simulink model "FrequencySupport_OSC1_or_OSC2"  (R2022a)
settings: Solver=ode15s  StartTime=0.0  StopTime=50  RelTol=1e-3
model workspace (MAT data in the model file):
  Cdc = 0.05
  c_dc = 0.05
values from neighbouring files (symbols this model uses):
  P_dis_bat = [9604.62056476 1369.7268469 1306.14940083 1303.28868815 1261.92740103 1202.52269752 1169.74670515 1107.03788784 1057.53947406 962.184427064 965.562157323 899.489129709 ... (3456 elements, 1152x3)]    [result_base.mat]
undefined symbols (not defined in the file or in its folder): C, D, f0, H_rec, H_send, Hvirt_BES, Hvirt_PV, K_bat_vir, Kf_BES, Kf_dc, Kf_EL, Kf_PV, Kf_WT, OC_HVDC, P_EL_0, P_load_vsc_rec, P_load_vsc_rec_2, P_PV_0, P_send_0, P_WT_0, Pdc0, R_down_bat, R_down_EL, R_down_PV, R_down_WT, R_PV_up_req, R_syn_rec, R_up_bat, R_up_EL, R_up_PV, R_up_WT, R_WT_up_req, S_BES, S_EL, S_HVDC, S_PV, S_rec, S_rec_hydra, S_rec_syn, S_send, S_send_syn, S_WT, Sliding_window_t, T_ch, T_g_syn, T_g_w, T_rh, T_w
settings Model: Creator=Douzi  LastModifiedBy=Douzi

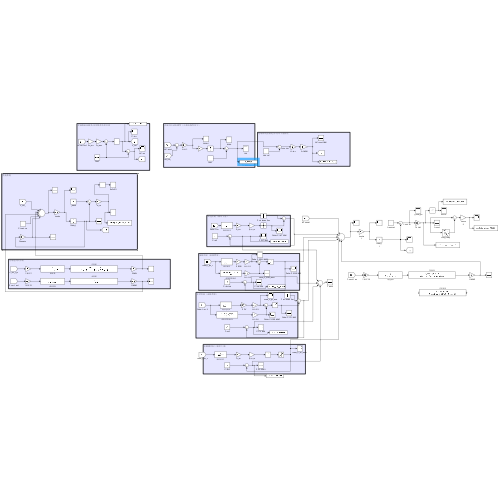
[thumbnail: Simulink's stored preview of the top-level diagram]
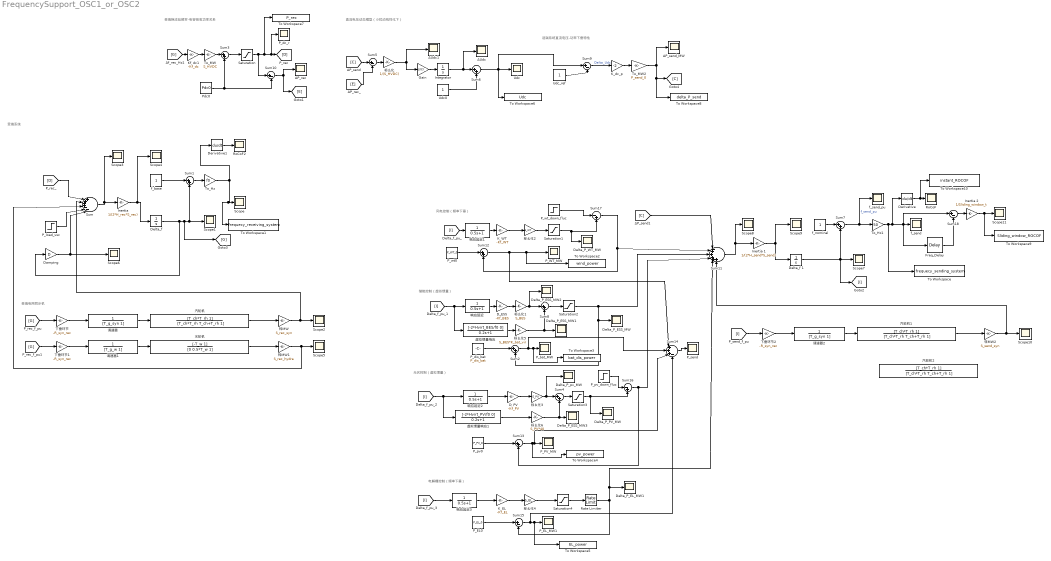
== system FrequencySupport_OSC1_or_OSC2 ==
  note: 受端电网同步机
  note: 储能控制（虚拟惯量）
  note: 风电控制（频率下垂）
  note: 受端换流站频率-电容吸收功率关系
  note: 受端系统
  note: 光伏控制（虚拟惯量）
  note: 电解槽控制（频率下垂）
  note: 直流电压动态模型（小扰动线性化下）
  note: 送端系统直流电压-功率下垂特性
  D_ESS : Gain  Gain=-Kf_BES
  D_PV : Gain  Gain=-Kf_PV
  Damping : Gain  Gain=D
  Delta_P_EL_MW1 : Scope
  Delta_P_ESS_MW{,1..3} (4 alike) : Scope
  Delta_P_PV_MW : Scope
  Delta_P_WT_MW : Scope
  Delta_P_pv_MW : Scope
  "Delta_f " : Integrator
  Delta_f 1 : Integrator
  Derivative : Derivative
  Derivative1 : Derivative
  Freq_Delay : TransportDelay  DelayTime=Sliding_window_t  InitialOutput=50
  Gain : Gain  Gain=1/(C)
  "Inertia " : Gain  Gain=1/(2*H_rec*S_rec)
  Inertia 1 : Gain  Gain=1/(2*H_send*S_send)
  Inertia 2 : Gain  Gain=1/Sliding_window_t
  Integrator : Integrator
  K_EL : Gain  Gain=-Kf_EL
  K_WT : Gain  Gain=-Kf_WT
  K_dc_p : Gain  Gain=-2
  Kf_dc1 : Gain  Gain=-Kf_dc
  P_EL0 : Constant  Value=P_EL_0
  P_EL_MW1 : Scope
  P_PV_MW : Scope
  P_WT_MW : Scope
  P_bat_MW : Scope
  P_dc_r : Scope
  P_dis_bat : Constant  Value=P_dis_bat
  P_load_vsc : Step  Before=P_load_vsc_rec  After=P_load_vsc_rec_2  SampleTime=0
  P_pv0 : Constant  Value=P_PV_0
  P_pv_down_fluc : Step  After=R_PV_up_req  SampleTime=0
  P_send : Scope
  P_wt0 : Constant  Value=P_WT_0
  P_wt_down_fluc : Step  After=R_WT_up_req  SampleTime=0
  Pdc0 : Constant  Value=Pdc0
  Rate Limiter : RateLimiter  RisingSlewLimit=0.2*S_EL  FallingSlewLimit=-0.2*S_EL  SampleTimeMode=inherited
  RoCoF : Scope
  RoCoF2 : Scope
  Saturation : Saturate  UpperLimit=S_HVDC*OC_HVDC  LowerLimit=0
  Saturation1 : Saturate  UpperLimit=R_up_WT  LowerLimit=-R_down_WT
  Saturation2 : Saturate  UpperLimit=R_up_bat  LowerLimit=-R_down_bat
  Saturation3 : Saturate  UpperLimit=R_up_PV  LowerLimit=-R_down_PV
  Saturation4 : Saturate  UpperLimit=R_up_EL  LowerLimit=-R_down_EL
  Scope{,1..11} (12 alike) : Scope
  Sum : Sum  Inputs=|++++--|
  Sum{1..4,6..8,12..13} (9 alike) : Sum  Inputs=|++
  Sum{5,9..10,15,18} (5 alike) : Sum  Inputs=|+-
  Sum11 : Sum  Inputs=|-+++++
  Sum14 : Sum  Inputs=|+++-
  Sum16 : Sum  Inputs=|-+
  Sum17 : Sum  Inputs=|-+
  To Workspace : ToWorkspace  VariableName=frequecy_sending_system  SaveFormat=Structure With Time  SampleTime=-1
  To Workspace1 : ToWorkspace  VariableName=frequecy_receiving_system  SaveFormat=Structure With Time  SampleTime=-1
  To Workspace10 : ToWorkspace  VariableName=instant_ROCOF  SaveFormat=Structure With Time  SampleTime=-1
  To Workspace2 : ToWorkspace  VariableName=wind_power  SaveFormat=Structure With Time  SampleTime=-1
  To Workspace3 : ToWorkspace  VariableName=bat_dis_power  SaveFormat=Structure With Time  SampleTime=-1
  To Workspace4 : ToWorkspace  VariableName=pv_power  SaveFormat=Structure With Time  SampleTime=-1
  To Workspace5 : ToWorkspace  VariableName=EL_power  SaveFormat=Structure With Time  SampleTime=-1
  To Workspace6 : ToWorkspace  VariableName=Udc  SaveFormat=Structure With Time  SampleTime=-1
  To Workspace7 : ToWorkspace  VariableName=P_rec  SaveFormat=Structure With Time  SampleTime=-1
  To Workspace8 : ToWorkspace  VariableName=delta_P_send  SaveFormat=Structure With Time  SampleTime=-1
  To Workspace9 : ToWorkspace  VariableName=Sliding_window_ROCOF  SaveFormat=Structure With Time  SampleTime=-1
  To_Hz : Gain  Gain=f0
  To_Hz1 : Gain  Gain=50
  To_MW : Gain  Gain=S_HVDC
  To_MW2 : Gain  Gain=P_send_0
  Udc : Scope
  Udc0 : Constant
  Udc_ref : Constant
  f_base : Constant
  f_nominal : Constant
  f_send : Scope
  f_send_pu : Scope
  ΔP_rec : Scope
  ΔP_send_MW : Scope
  ΔUdc : Scope
  ΔUdc1 : Scope
  下垂环节 : Gain  Gain=-R_syn_rec
  下垂环节1 : Gain  Gain=-R_syn_rec
  下垂环节2 : Gain  Gain=-R_syn_rec
  响应延迟{,1..3} (4 alike) : TransferFcn  Denominator=[0.5 1]
  标幺化 : Gain  Gain=1/(S_HVDC)
  标幺化1 : Gain  Gain=S_BES
  标幺化2 : Gain  Gain=S_WT
  标幺化3 : Gain  Gain=S_PV
  标幺化4 : Gain  Gain=S_EL
  标幺化5 : Gain  Gain=S_BES*K_bat_vir
  标幺化6 : Gain  Gain=S_PV*40
  水轮机 : TransferFcn  Tag=汽轮机  Numerator=[-T_w 1]  Denominator=[0 0.5*T_w 1]
  汽轮机 : TransferFcn  Tag=汽轮机  Numerator=[T_ch*T_rh 1]  Denominator=[T_ch*T_rh T_ch+T_rh 1]
  汽轮机1 : TransferFcn  Tag=汽轮机  Numerator=[T_ch*T_rh 1]  Denominator=[T_ch*T_rh T_ch+T_rh 1]
  汽轮机2 : TransferFcn  Tag=汽轮机  Numerator=[T_ch*T_rh 1]  Denominator=[T_ch*T_rh T_ch+T_rh 1]
  虚拟惯量响应 : TransferFcn  Numerator=[-2*Hvirt_BES/f0 0]  Denominator=[0.2 1]
  虚拟惯量响应1 : TransferFcn  Numerator=[-2*Hvirt_PV/f0 0]  Denominator=[0.2 1]
  调速器 : TransferFcn  Denominator=[T_g_syn 1]
  调速器1 : TransferFcn  Denominator=[T_g_w 1]
  调速器2 : TransferFcn  Denominator=[T_g_syn 1]
  转MW : Gain  Gain=S_rec_syn
  转MW1 : Gain  Gain=S_rec_hydra
  转MW2 : Gain  Gain=S_send_syn
  wires:
  P_load_vsc/1 -> Sum/5
  Sum/1 -> Scope3/1, "Inertia "/1
  "Inertia "/1 -> Scope4/1, "Delta_f "/1
  "Delta_f "/1 -> [G], Scope1/1, Sum1/2, Damping/1
  f_base/1 -> Sum1/1
  Sum1/1 -> To_Hz/1
  Damping/1 -> Scope6/1, Sum/6
  To_Hz/1 -> To Workspace1/1, Scope/1, Derivative1/1
  Pdc0/1 -> Sum10/2, Sum3/2
  Sum3/1 -> Saturation/1
  Saturation/1 -> Sum10/1, P_dc_r/1, [D], To Workspace7/1
  f_nominal/1 -> Sum7/1
  Sum7/1 -> f_send_pu/1, To_Hz1/1  "f_send_pu"
  To_Hz1/1 -> Derivative/1, Sum18/1, Freq_Delay/1, f_send/1, To Workspace/1
  Saturation1/1 -> Sum17/2, Delta_P_WT_MW/1
  Derivative/1 -> To Workspace10/1, RoCoF/1
  [I] -> 虚拟惯量响应1/1, 响应延迟2/1
  Saturation3/1 -> Sum16/2, Delta_P_PV_MW/1
  [D] -> Sum/2
  Sum10/1 -> ΔP_rec/1, [E]
  K_WT/1 -> 标幺化2/1
  标幺化2/1 -> Saturation1/1
  [G] -> 下垂环节/1
  下垂环节/1 -> 调速器/1
  调速器/1 -> 汽轮机/1
  汽轮机/1 -> 转MW/1
  转MW/1 -> Sum/3, Scope2/1
  下垂环节1/1 -> 调速器1/1
  调速器1/1 -> 水轮机/1
  水轮机/1 -> 转MW1/1
  [G] -> 下垂环节1/1
  转MW1/1 -> Scope5/1, Sum/4
  [G] -> Kf_dc1/1
  Kf_dc1/1 -> To_MW/1
  To_MW/1 -> Sum3/1
  P_wt0/1 -> Sum12/1
  Sum12/1 -> Sum14/1, To Workspace2/1, P_WT_MW/1
  P_dis_bat/1 -> Sum2/1
  Sum2/1 -> Sum14/2, To Workspace3/1, P_bat_MW/1
  Saturation2/1 -> Sum11/3, Delta_P_ESS_MW/1, Sum2/2
  P_pv0/1 -> Sum13/1
  Sum13/1 -> To Workspace4/1, Sum14/3, P_PV_MW/1
  Sum14/1 -> P_send/1
  标幺化4/1 -> Saturation4/1
  Sum15/1 -> Sum14/4, To Workspace5/1, P_EL_MW1/1
  P_EL0/1 -> Sum15/1
  Saturation4/1 -> Rate Limiter/1
  K_EL/1 -> 标幺化4/1
  [I] -> 响应延迟3/1
  Rate Limiter/1 -> Sum11/5, Delta_P_EL_MW1/1, Sum15/2
  Derivative1/1 -> RoCoF2/1
  Delta_f 1/1 -> Scope7/1, [I], Sum7/2
  Sum11/1 -> Scope8/1, Inertia 1/1
  Inertia 1/1 -> Scope9/1, Delta_f 1/1
  下垂环节2/1 -> 调速器2/1
  调速器2/1 -> 汽轮机1/1
  [I] -> 下垂环节2/1
  转MW2/1 -> Sum11/6, Scope10/1
  汽轮机1/1 -> 转MW2/1
  [I] -> 虚拟惯量响应/1, 响应延迟/1
  响应延迟/1 -> D_ESS/1
  D_ESS/1 -> 标幺化1/1
  虚拟惯量响应/1 -> 标幺化5/1
  标幺化1/1 -> Delta_P_ESS_MW2/1, Sum8/1
  标幺化5/1 -> Sum8/2, Delta_P_ESS_MW1/1
  Sum8/1 -> Saturation2/1
  [I] -> 响应延迟1/1
  响应延迟1/1 -> K_WT/1
  虚拟惯量响应1/1 -> 标幺化6/1
  响应延迟2/1 -> D_PV/1
  D_PV/1 -> 标幺化3/1
  标幺化3/1 -> Sum4/1, Delta_P_pv_MW/1
  Sum4/1 -> Saturation3/1
  标幺化6/1 -> Sum4/2, Delta_P_ESS_MW3/1
  响应延迟3/1 -> K_EL/1
  标幺化/1 -> ΔUdc1/1, Gain/1
  Integrator/1 -> Sum6/1, ΔUdc/1
  Sum6/1 -> To Workspace6/1, Sum9/1, Udc/1
  Udc0/1 -> Sum6/2
  [C] -> Sum5/1
  Sum5/1 -> 标幺化/1
  [E] -> Sum5/2
  Gain/1 -> Integrator/1
  To_MW2/1 -> To Workspace8/1, [C], ΔP_send_MW/1
  Sum9/1 -> K_dc_p/1  "Delta_Udc"
  Udc_ref/1 -> Sum9/2
  K_dc_p/1 -> To_MW2/1
  [C] -> Sum11/1
  P_pv_down_fluc/1 -> Sum16/1
  Sum16/1 -> Sum13/2, Sum11/4
  P_wt_down_fluc/1 -> Sum17/1
  Sum17/1 -> Sum12/2, Sum11/2
  Freq_Delay/1 -> Sum18/2
  Sum18/1 -> Inertia 2/1
  Inertia 2/1 -> To Workspace9/1, Scope11/1
